simulink subsystem "Piero_HW"  (R2023b)
settings: Solver=VariableStepAuto  StartTime=0.0  StopTime=10.0  RelTol=1e-3
libraries: simulink x2
settings Model: Creator=Enrique  LastModifiedBy=Enrique

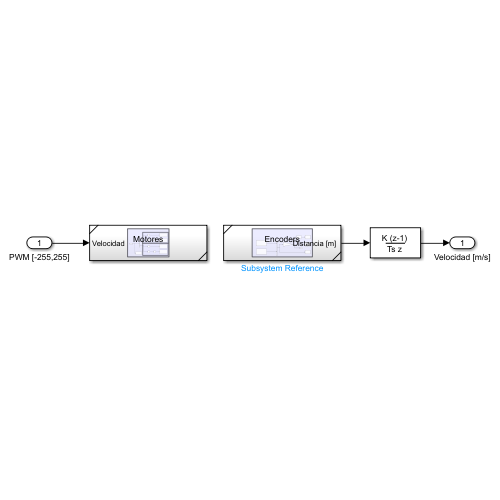
[thumbnail: Simulink's stored preview of the top-level diagram]
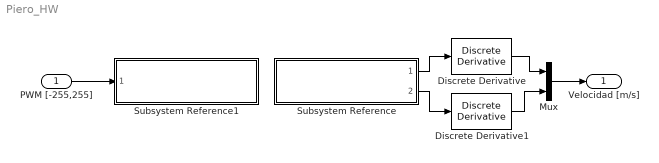
== system Piero_HW ==
  PWM [-255,255] : Inport
  Discrete Derivative : simulink/Discrete/Discrete Derivative  gainval=1.0  ICPrevScaledInput=0.0  OutMin=[]  OutMax=[]  OutDataType=fixdt(1, 16)  OutScaling=2^-10  DoSatur=off
  Discrete Derivative1 : simulink/Discrete/Discrete Derivative  gainval=1.0  ICPrevScaledInput=0.0  OutMin=[]  OutMax=[]  OutDataType=fixdt(1, 16)  OutScaling=2^-10  DoSatur=off
  Mux : Mux  Inputs=2
  Subsystem Reference : Subsystem  ReferencedSubsystem=Encoders
  Subsystem Reference1 : Subsystem  ReferencedSubsystem=Motores
  Velocidad [m/s] : Outport
  wires:
  PWM [-255,255]/1 -> Subsystem Reference1/1
  Subsystem Reference/1 -> Discrete Derivative/1
  Subsystem Reference/2 -> Discrete Derivative1/1
  Mux/1 -> Velocidad [m/s]/1
  Discrete Derivative1/1 -> Mux/2
  Discrete Derivative/1 -> Mux/1
